simulink model "pneumatic_tank_general_PI_R2018a"  (R2018a)
settings: Solver=ode15s  StartTime=0.0  StopTime=20  RelTol=1e-4
model workspace (MATLAB code in the model file):
  | V = 0.4; %liter
  | alpha = 1.5/3;
  | p_s = 6; % bar
settings Model: Creator=kjartan  LastModifiedBy=kjartan
settings SFSimCC: SimUseLocalCustomCode=on
settings RTWCC: RTWUseLocalCustomCode=on

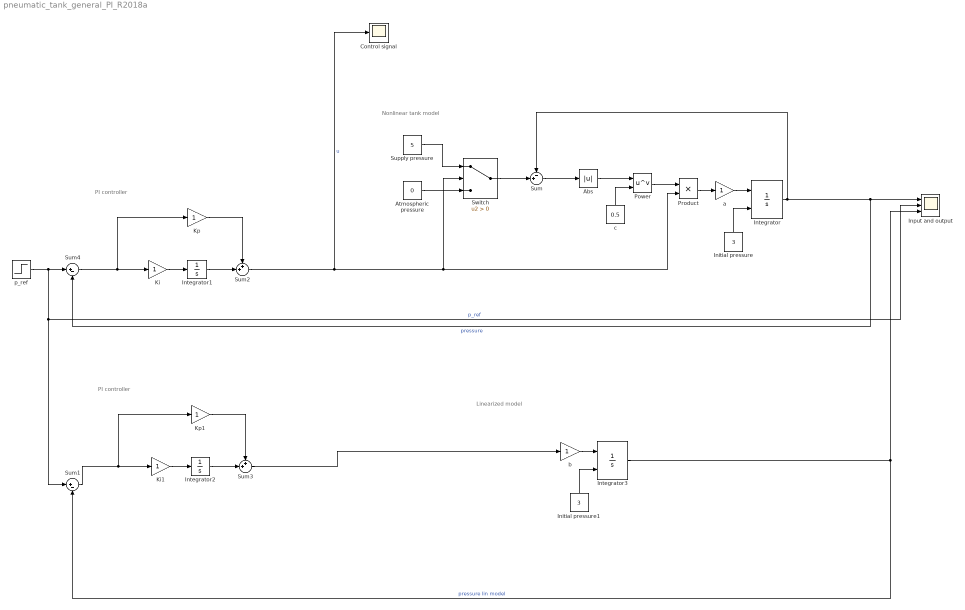
== system pneumatic_tank_general_PI_R2018a ==
  note: Linearized model
  note: PI controller
  note: Nonlinear tank model
  note: PI controller
  Abs : Abs
  Atmospheric pressure : Constant  Value=0
  Control signal : Scope
  Initial pressure : Constant  Value=3  OutDataTypeStr=Inherit: Inherit via back propagation
  Initial pressure1 : Constant  Value=3  OutDataTypeStr=Inherit: Inherit via back propagation
  Input and output : Scope  NumInputPorts=3
  Integrator : Integrator  InitialConditionSource=external  InitialCondition=1  LimitOutput=on  UpperSaturationLimit=5  LowerSaturationLimit=0
  Integrator1 : Integrator
  Integrator2 : Integrator
  Integrator3 : Integrator  InitialConditionSource=external  InitialCondition=1  LowerSaturationLimit=0
  Ki : Gain
  Ki1 : Gain
  Kp : Gain
  Kp1 : Gain
  Power : Math  Operator=pow  SaturateOnIntegerOverflow=on
  Product : Product
  Sum : Sum  Inputs=-+|
  Sum1 : Sum  Inputs=|+-
  Sum2 : Sum  Inputs=++|
  Sum3 : Sum  Inputs=++|
  Sum4 : Sum  Inputs=|+-
  Supply pressure : Constant  Value=5
  Switch : Switch  Criteria=u2 > Threshold
  a : Gain
  b : Gain
  c : Constant  Value=0.5
  p_ref : Step  Time=5  After=4  SampleTime=0
  wires:
  Integrator/1 -> Sum/1, Sum4/2, Input and output/1  "pressure"
  Sum/1 -> Abs/1
  Sum2/1 -> Control signal/1, Switch/2, Product/2  "u"
  a/1 -> Integrator/1
  Product/1 -> a/1
  Supply pressure/1 -> Switch/1
  Atmospheric pressure/1 -> Switch/3
  Switch/1 -> Sum/2
  Power/1 -> Product/1
  Initial pressure/1 -> Integrator/2
  Abs/1 -> Power/1
  c/1 -> Power/2
  Integrator1/1 -> Sum2/2
  Ki/1 -> Integrator1/1
  Kp/1 -> Sum2/1
  Ki1/1 -> Integrator2/1
  Sum3/1 -> b/1
  Kp1/1 -> Sum3/1
  Integrator2/1 -> Sum3/2
  Sum4/1 -> Kp/1, Ki/1
  p_ref/1 -> Sum1/1, Input and output/2, Sum4/1  "p_ref"
  b/1 -> Integrator3/1
  Initial pressure1/1 -> Integrator3/2
  Integrator3/1 -> Input and output/3, Sum1/2  "pressure lin model"
  Sum1/1 -> Kp1/1, Ki1/1
